simulink model "gm_DSBF"  (R2019b)
settings: Solver=FixedStepDiscrete  StartTime=0.0  StopTime=0.02  RelTol=1e-3
InitFcn:
  | sm_callback_init
StopFcn:
  | sm_callback_stop
undefined symbols (not defined in the file or in its folder): arraySize, arraySpacing, delayDataTypeFractionLength, delayDataTypeSign, delayDataTypeWordLength, mp, samplingRate, speedOfSound, upsampleFactor
libraries: hdlsllib x64, simulink x36, dspmlti4 x16, dsphdlfiltering x16
(part 2 of 5)

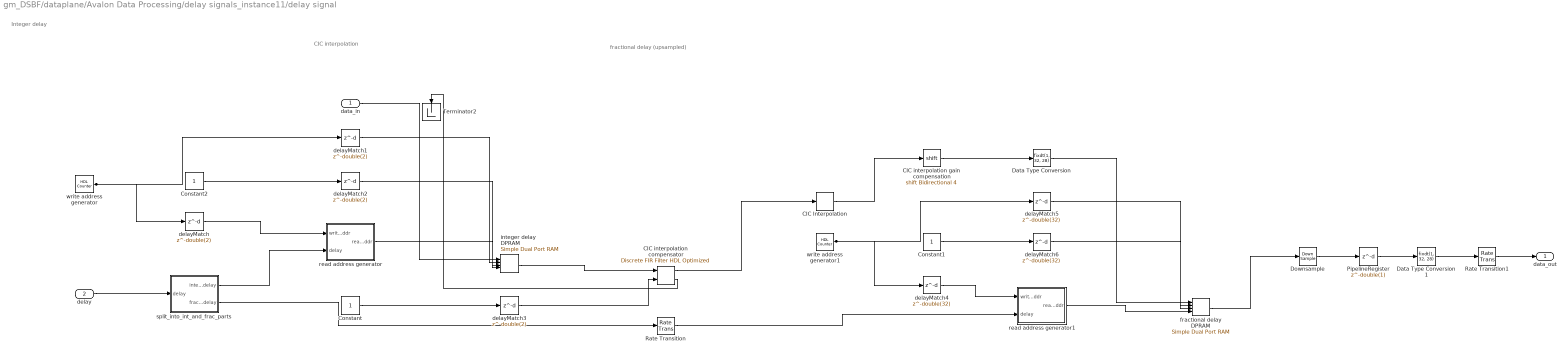
== system gm_DSBF/dataplane/Avalon Data Processing/delay signals_instance11/delay signal ==
  note: CIC interpolation
  note: Integer delay
  note: fractional delay (upsampled)
  data_in : Inport  OutDataTypeStr=fixdt(1, 32, 28)  PortDimensions=1  SampleTime=2.08333333333333e-05
  delay : Inport  Port=2  OutDataTypeStr=fixdt(1, 12, 6)  PortDimensions=1  SampleTime=2.08333333333333e-05
  CIC Interpolation : dspmlti4/CIC Interpolation  filtFrom=Filter object  filtobj=mp.cicInterpolator  ftype=Interpolator  R=mp.upsampleFactor  M=1  N=2  filterInternals=Full precision  BPS=[16 16 16 16]  FLPS=0  outputWordLength=32  outputFracLength=0  launchFVT=off  framing=Allow multirate processing  OutputFrames=off
      settings: SourceProductName=DSP System Toolbox  SourceProductBaseCode=DS
  CIC interpolation compensator : dsphdlfiltering/Discrete FIR Filter HDL Optimized  NumeratorSource=Property  Numerator=mp.cicInterpolatorCompensator.coeffs.Numerator  NumeratorPrototype=[]  FilterStructure=Direct form systolic  SerializationOption=Maximum number of multipliers  NumberOfCycles=2  NumberOfMultipliers=4  SimulateUsing=Code generation  roundingMode=Floor  overflowMode=off  CoefficientsDataTypeStr=fixdt(1,16)  CoefficientsMin=[]  CoefficientsMax=[]  OutputDataTypeStr=Inherit: Same word length as input  OutputMin=[]  OutputMax=[]  ResetInputPort=off  HDLGlobalReset=off
      settings: SourceProductName=DSP System Toolbox  SourceProductBaseCode=DS
  CIC interpolation gain compensation : ArithShift  BitShiftNumber=4  BinPtShiftNumber=double(0)
  Constant : Constant  OutDataTypeStr=boolean  SampleTime=-1
  Constant1 : Constant  OutDataTypeStr=boolean  SampleTime=-1
  Constant2 : Constant  OutDataTypeStr=boolean  SampleTime=-1
  Data Type Conversion : DataTypeConversion  OutDataTypeStr=fixdt(1, 32, 28)  SampleTime=1.30208333333333e-06
  Data Type Conversion1 : DataTypeConversion  OutDataTypeStr=fixdt(1, 32, 28)  SampleTime=2.08333333333333e-05
  Downsample : DownSample  N=double(16)  phase=double(0)  RateOptions=Allow multirate processing
  PipelineRegister : Delay  DelayLength=double(1)  InitialCondition=0  SampleTime=2.08333333333333e-05
  Rate Transition : RateTransition  InitialCondition=double(0)  OutPortSampleTimeOpt=Multiple of input port sample time  OutPortSampleTimeMultiple=1/16
  Rate Transition1 : RateTransition  InitialCondition=double(0)  OutPortSampleTimeOpt=Multiple of input port sample time  OutPortSampleTimeMultiple=1/2048
  Terminator2 : Terminator
  delayMatch{,1..3} (4 alike) : Delay  DelayLength=double(2)  InitialCondition=0  SampleTime=2.08333333333333e-05
  delayMatch4 : Delay  DelayLength=double(32)  InitialCondition=0  SampleTime=1.30208333333333e-06
  delayMatch5 : Delay  DelayLength=double(32)  InitialCondition=0  SampleTime=1.30208333333333e-06
  delayMatch6 : Delay  DelayLength=double(32)  InitialCondition=0  SampleTime=1.30208333333333e-06
  fractional delay DPRAM : hdlsllib/HDL RAMs/Simple Dual Port RAM  ram_size=mp.fractionalDelayAddrSize
      settings: SourceProductName=Simulink  SourceProductBaseCode=SL
  integer delay DPRAM : hdlsllib/HDL RAMs/Simple Dual Port RAM  ram_size=mp.integerDelayAddrSize
      settings: SourceProductName=Simulink  SourceProductBaseCode=SL
  read address generator : Subsystem
  read address generator1 : Subsystem
  split_into_int_and_frac_parts : Subsystem
  write address generator : hdlsllib/Sources/HDL Counter  CountType=Count limited  CountInit=double(0)  CountStep=double(1)  CountMax=double(63)  CountFromType=Initial value  CountFrom=double(0)  CountResetPort=off  CountLoadPort=off  CountEnbPort=off  CountDirPort=off  CountDataType=Unsigned  CountWordLen=6  CountFracLen=0  CountSampTime=2.08333333333333e-05
      settings: SourceProductName=Simulink
  write address generator1 : hdlsllib/Sources/HDL Counter  CountType=Count limited  CountInit=double(0)  CountStep=double(1)  CountMax=double(63)  CountFromType=Initial value  CountFrom=double(0)  CountResetPort=off  CountLoadPort=off  CountEnbPort=off  CountDirPort=off  CountDataType=Unsigned  CountWordLen=6  CountFracLen=0  CountSampTime=1.30208333333333e-06
      settings: SourceProductName=Simulink
  data_out : Outport  VectorParamsAs1DForOutWhenUnconnected=off
  wires:
  Downsample/1 -> PipelineRegister/1
  CIC interpolation gain compensation/1 -> Data Type Conversion/1
  split_into_int_and_frac_parts/1(integer_delay) -> read address generator/2(delay)
  Constant1/1 -> delayMatch6/1
  write address generator1/1 -> delayMatch4/1, delayMatch5/1
  delayMatch5/1 -> fractional delay DPRAM/2
  Constant/1 -> delayMatch3/1
  Constant2/1 -> delayMatch2/1
  write address generator/1 -> delayMatch/1, delayMatch1/1
  delayMatch1/1 -> integer delay DPRAM/2
  delay/1 -> split_into_int_and_frac_parts/1(delay)
  data_in/1 -> integer delay DPRAM/1
  delayMatch3/1 -> CIC interpolation compensator/2
  delayMatch6/1 -> fractional delay DPRAM/3
  delayMatch2/1 -> integer delay DPRAM/3
  Data Type Conversion/1 -> fractional delay DPRAM/1
  Data Type Conversion1/1 -> Rate Transition1/1
  split_into_int_and_frac_parts/2(fractional_delay) -> Rate Transition/1
  read address generator/1(read_addr) -> integer delay DPRAM/4
  read address generator1/1(read_addr) -> fractional delay DPRAM/4
  CIC Interpolation/1 -> CIC interpolation gain compensation/1
  CIC interpolation compensator/2 -> Terminator2/1
  CIC interpolation compensator/1 -> CIC Interpolation/1
  PipelineRegister/1 -> Data Type Conversion1/1
  Rate Transition/1 -> read address generator1/2(delay)
  Rate Transition1/1 -> data_out/1
  fractional delay DPRAM/1 -> Downsample/1
  integer delay DPRAM/1 -> CIC interpolation compensator/1
  delayMatch/1 -> read address generator/1(write_addr)
  delayMatch4/1 -> read address generator1/1(write_addr)

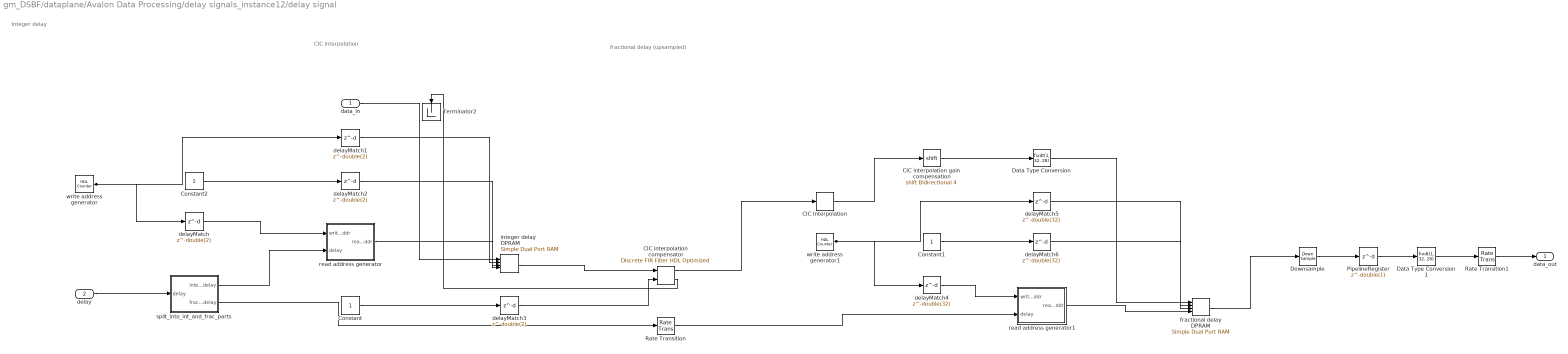
== system gm_DSBF/dataplane/Avalon Data Processing/delay signals_instance12/delay signal ==
  note: CIC interpolation
  note: Integer delay
  note: fractional delay (upsampled)
  data_in : Inport  OutDataTypeStr=fixdt(1, 32, 28)  PortDimensions=1  SampleTime=2.08333333333333e-05
  delay : Inport  Port=2  OutDataTypeStr=fixdt(1, 12, 6)  PortDimensions=1  SampleTime=2.08333333333333e-05
  CIC Interpolation : dspmlti4/CIC Interpolation  filtFrom=Filter object  filtobj=mp.cicInterpolator  ftype=Interpolator  R=mp.upsampleFactor  M=1  N=2  filterInternals=Full precision  BPS=[16 16 16 16]  FLPS=0  outputWordLength=32  outputFracLength=0  launchFVT=off  framing=Allow multirate processing  OutputFrames=off
      settings: SourceProductName=DSP System Toolbox  SourceProductBaseCode=DS
  CIC interpolation compensator : dsphdlfiltering/Discrete FIR Filter HDL Optimized  NumeratorSource=Property  Numerator=mp.cicInterpolatorCompensator.coeffs.Numerator  NumeratorPrototype=[]  FilterStructure=Direct form systolic  SerializationOption=Maximum number of multipliers  NumberOfCycles=2  NumberOfMultipliers=4  SimulateUsing=Code generation  roundingMode=Floor  overflowMode=off  CoefficientsDataTypeStr=fixdt(1,16)  CoefficientsMin=[]  CoefficientsMax=[]  OutputDataTypeStr=Inherit: Same word length as input  OutputMin=[]  OutputMax=[]  ResetInputPort=off  HDLGlobalReset=off
      settings: SourceProductName=DSP System Toolbox  SourceProductBaseCode=DS
  CIC interpolation gain compensation : ArithShift  BitShiftNumber=4  BinPtShiftNumber=double(0)
  Constant : Constant  OutDataTypeStr=boolean  SampleTime=-1
  Constant1 : Constant  OutDataTypeStr=boolean  SampleTime=-1
  Constant2 : Constant  OutDataTypeStr=boolean  SampleTime=-1
  Data Type Conversion : DataTypeConversion  OutDataTypeStr=fixdt(1, 32, 28)  SampleTime=1.30208333333333e-06
  Data Type Conversion1 : DataTypeConversion  OutDataTypeStr=fixdt(1, 32, 28)  SampleTime=2.08333333333333e-05
  Downsample : DownSample  N=double(16)  phase=double(0)  RateOptions=Allow multirate processing
  PipelineRegister : Delay  DelayLength=double(1)  InitialCondition=0  SampleTime=2.08333333333333e-05
  Rate Transition : RateTransition  InitialCondition=double(0)  OutPortSampleTimeOpt=Multiple of input port sample time  OutPortSampleTimeMultiple=1/16
  Rate Transition1 : RateTransition  InitialCondition=double(0)  OutPortSampleTimeOpt=Multiple of input port sample time  OutPortSampleTimeMultiple=1/2048
  Terminator2 : Terminator
  delayMatch{,1..3} (4 alike) : Delay  DelayLength=double(2)  InitialCondition=0  SampleTime=2.08333333333333e-05
  delayMatch4 : Delay  DelayLength=double(32)  InitialCondition=0  SampleTime=1.30208333333333e-06
  delayMatch5 : Delay  DelayLength=double(32)  InitialCondition=0  SampleTime=1.30208333333333e-06
  delayMatch6 : Delay  DelayLength=double(32)  InitialCondition=0  SampleTime=1.30208333333333e-06
  fractional delay DPRAM : hdlsllib/HDL RAMs/Simple Dual Port RAM  ram_size=mp.fractionalDelayAddrSize
      settings: SourceProductName=Simulink  SourceProductBaseCode=SL
  integer delay DPRAM : hdlsllib/HDL RAMs/Simple Dual Port RAM  ram_size=mp.integerDelayAddrSize
      settings: SourceProductName=Simulink  SourceProductBaseCode=SL
  read address generator : Subsystem
  read address generator1 : Subsystem
  split_into_int_and_frac_parts : Subsystem
  write address generator : hdlsllib/Sources/HDL Counter  CountType=Count limited  CountInit=double(0)  CountStep=double(1)  CountMax=double(63)  CountFromType=Initial value  CountFrom=double(0)  CountResetPort=off  CountLoadPort=off  CountEnbPort=off  CountDirPort=off  CountDataType=Unsigned  CountWordLen=6  CountFracLen=0  CountSampTime=2.08333333333333e-05
      settings: SourceProductName=Simulink
  write address generator1 : hdlsllib/Sources/HDL Counter  CountType=Count limited  CountInit=double(0)  CountStep=double(1)  CountMax=double(63)  CountFromType=Initial value  CountFrom=double(0)  CountResetPort=off  CountLoadPort=off  CountEnbPort=off  CountDirPort=off  CountDataType=Unsigned  CountWordLen=6  CountFracLen=0  CountSampTime=1.30208333333333e-06
      settings: SourceProductName=Simulink
  data_out : Outport  VectorParamsAs1DForOutWhenUnconnected=off
  wires:
  Downsample/1 -> PipelineRegister/1
  CIC interpolation gain compensation/1 -> Data Type Conversion/1
  split_into_int_and_frac_parts/1(integer_delay) -> read address generator/2(delay)
  Constant1/1 -> delayMatch6/1
  write address generator1/1 -> delayMatch4/1, delayMatch5/1
  delayMatch5/1 -> fractional delay DPRAM/2
  Constant/1 -> delayMatch3/1
  Constant2/1 -> delayMatch2/1
  write address generator/1 -> delayMatch/1, delayMatch1/1
  delayMatch1/1 -> integer delay DPRAM/2
  delay/1 -> split_into_int_and_frac_parts/1(delay)
  data_in/1 -> integer delay DPRAM/1
  delayMatch3/1 -> CIC interpolation compensator/2
  delayMatch6/1 -> fractional delay DPRAM/3
  delayMatch2/1 -> integer delay DPRAM/3
  Data Type Conversion/1 -> fractional delay DPRAM/1
  Data Type Conversion1/1 -> Rate Transition1/1
  split_into_int_and_frac_parts/2(fractional_delay) -> Rate Transition/1
  read address generator/1(read_addr) -> integer delay DPRAM/4
  read address generator1/1(read_addr) -> fractional delay DPRAM/4
  CIC Interpolation/1 -> CIC interpolation gain compensation/1
  CIC interpolation compensator/2 -> Terminator2/1
  CIC interpolation compensator/1 -> CIC Interpolation/1
  PipelineRegister/1 -> Data Type Conversion1/1
  Rate Transition/1 -> read address generator1/2(delay)
  Rate Transition1/1 -> data_out/1
  fractional delay DPRAM/1 -> Downsample/1
  integer delay DPRAM/1 -> CIC interpolation compensator/1
  delayMatch/1 -> read address generator/1(write_addr)
  delayMatch4/1 -> read address generator1/1(write_addr)

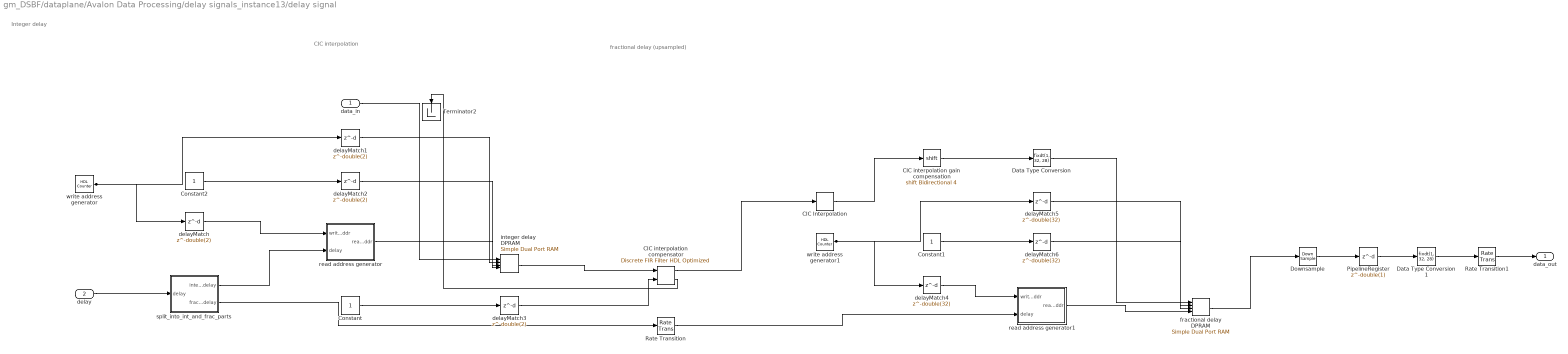
== system gm_DSBF/dataplane/Avalon Data Processing/delay signals_instance13/delay signal ==
  note: CIC interpolation
  note: Integer delay
  note: fractional delay (upsampled)
  data_in : Inport  OutDataTypeStr=fixdt(1, 32, 28)  PortDimensions=1  SampleTime=2.08333333333333e-05
  delay : Inport  Port=2  OutDataTypeStr=fixdt(1, 12, 6)  PortDimensions=1  SampleTime=2.08333333333333e-05
  CIC Interpolation : dspmlti4/CIC Interpolation  filtFrom=Filter object  filtobj=mp.cicInterpolator  ftype=Interpolator  R=mp.upsampleFactor  M=1  N=2  filterInternals=Full precision  BPS=[16 16 16 16]  FLPS=0  outputWordLength=32  outputFracLength=0  launchFVT=off  framing=Allow multirate processing  OutputFrames=off
      settings: SourceProductName=DSP System Toolbox  SourceProductBaseCode=DS
  CIC interpolation compensator : dsphdlfiltering/Discrete FIR Filter HDL Optimized  NumeratorSource=Property  Numerator=mp.cicInterpolatorCompensator.coeffs.Numerator  NumeratorPrototype=[]  FilterStructure=Direct form systolic  SerializationOption=Maximum number of multipliers  NumberOfCycles=2  NumberOfMultipliers=4  SimulateUsing=Code generation  roundingMode=Floor  overflowMode=off  CoefficientsDataTypeStr=fixdt(1,16)  CoefficientsMin=[]  CoefficientsMax=[]  OutputDataTypeStr=Inherit: Same word length as input  OutputMin=[]  OutputMax=[]  ResetInputPort=off  HDLGlobalReset=off
      settings: SourceProductName=DSP System Toolbox  SourceProductBaseCode=DS
  CIC interpolation gain compensation : ArithShift  BitShiftNumber=4  BinPtShiftNumber=double(0)
  Constant : Constant  OutDataTypeStr=boolean  SampleTime=-1
  Constant1 : Constant  OutDataTypeStr=boolean  SampleTime=-1
  Constant2 : Constant  OutDataTypeStr=boolean  SampleTime=-1
  Data Type Conversion : DataTypeConversion  OutDataTypeStr=fixdt(1, 32, 28)  SampleTime=1.30208333333333e-06
  Data Type Conversion1 : DataTypeConversion  OutDataTypeStr=fixdt(1, 32, 28)  SampleTime=2.08333333333333e-05
  Downsample : DownSample  N=double(16)  phase=double(0)  RateOptions=Allow multirate processing
  PipelineRegister : Delay  DelayLength=double(1)  InitialCondition=0  SampleTime=2.08333333333333e-05
  Rate Transition : RateTransition  InitialCondition=double(0)  OutPortSampleTimeOpt=Multiple of input port sample time  OutPortSampleTimeMultiple=1/16
  Rate Transition1 : RateTransition  InitialCondition=double(0)  OutPortSampleTimeOpt=Multiple of input port sample time  OutPortSampleTimeMultiple=1/2048
  Terminator2 : Terminator
  delayMatch{,1..3} (4 alike) : Delay  DelayLength=double(2)  InitialCondition=0  SampleTime=2.08333333333333e-05
  delayMatch4 : Delay  DelayLength=double(32)  InitialCondition=0  SampleTime=1.30208333333333e-06
  delayMatch5 : Delay  DelayLength=double(32)  InitialCondition=0  SampleTime=1.30208333333333e-06
  delayMatch6 : Delay  DelayLength=double(32)  InitialCondition=0  SampleTime=1.30208333333333e-06
  fractional delay DPRAM : hdlsllib/HDL RAMs/Simple Dual Port RAM  ram_size=mp.fractionalDelayAddrSize
      settings: SourceProductName=Simulink  SourceProductBaseCode=SL
  integer delay DPRAM : hdlsllib/HDL RAMs/Simple Dual Port RAM  ram_size=mp.integerDelayAddrSize
      settings: SourceProductName=Simulink  SourceProductBaseCode=SL
  read address generator : Subsystem
  read address generator1 : Subsystem
  split_into_int_and_frac_parts : Subsystem
  write address generator : hdlsllib/Sources/HDL Counter  CountType=Count limited  CountInit=double(0)  CountStep=double(1)  CountMax=double(63)  CountFromType=Initial value  CountFrom=double(0)  CountResetPort=off  CountLoadPort=off  CountEnbPort=off  CountDirPort=off  CountDataType=Unsigned  CountWordLen=6  CountFracLen=0  CountSampTime=2.08333333333333e-05
      settings: SourceProductName=Simulink
  write address generator1 : hdlsllib/Sources/HDL Counter  CountType=Count limited  CountInit=double(0)  CountStep=double(1)  CountMax=double(63)  CountFromType=Initial value  CountFrom=double(0)  CountResetPort=off  CountLoadPort=off  CountEnbPort=off  CountDirPort=off  CountDataType=Unsigned  CountWordLen=6  CountFracLen=0  CountSampTime=1.30208333333333e-06
      settings: SourceProductName=Simulink
  data_out : Outport  VectorParamsAs1DForOutWhenUnconnected=off
  wires:
  Downsample/1 -> PipelineRegister/1
  CIC interpolation gain compensation/1 -> Data Type Conversion/1
  split_into_int_and_frac_parts/1(integer_delay) -> read address generator/2(delay)
  Constant1/1 -> delayMatch6/1
  write address generator1/1 -> delayMatch4/1, delayMatch5/1
  delayMatch5/1 -> fractional delay DPRAM/2
  Constant/1 -> delayMatch3/1
  Constant2/1 -> delayMatch2/1
  write address generator/1 -> delayMatch/1, delayMatch1/1
  delayMatch1/1 -> integer delay DPRAM/2
  delay/1 -> split_into_int_and_frac_parts/1(delay)
  data_in/1 -> integer delay DPRAM/1
  delayMatch3/1 -> CIC interpolation compensator/2
  delayMatch6/1 -> fractional delay DPRAM/3
  delayMatch2/1 -> integer delay DPRAM/3
  Data Type Conversion/1 -> fractional delay DPRAM/1
  Data Type Conversion1/1 -> Rate Transition1/1
  split_into_int_and_frac_parts/2(fractional_delay) -> Rate Transition/1
  read address generator/1(read_addr) -> integer delay DPRAM/4
  read address generator1/1(read_addr) -> fractional delay DPRAM/4
  CIC Interpolation/1 -> CIC interpolation gain compensation/1
  CIC interpolation compensator/2 -> Terminator2/1
  CIC interpolation compensator/1 -> CIC Interpolation/1
  PipelineRegister/1 -> Data Type Conversion1/1
  Rate Transition/1 -> read address generator1/2(delay)
  Rate Transition1/1 -> data_out/1
  fractional delay DPRAM/1 -> Downsample/1
  integer delay DPRAM/1 -> CIC interpolation compensator/1
  delayMatch/1 -> read address generator/1(write_addr)
  delayMatch4/1 -> read address generator1/1(write_addr)

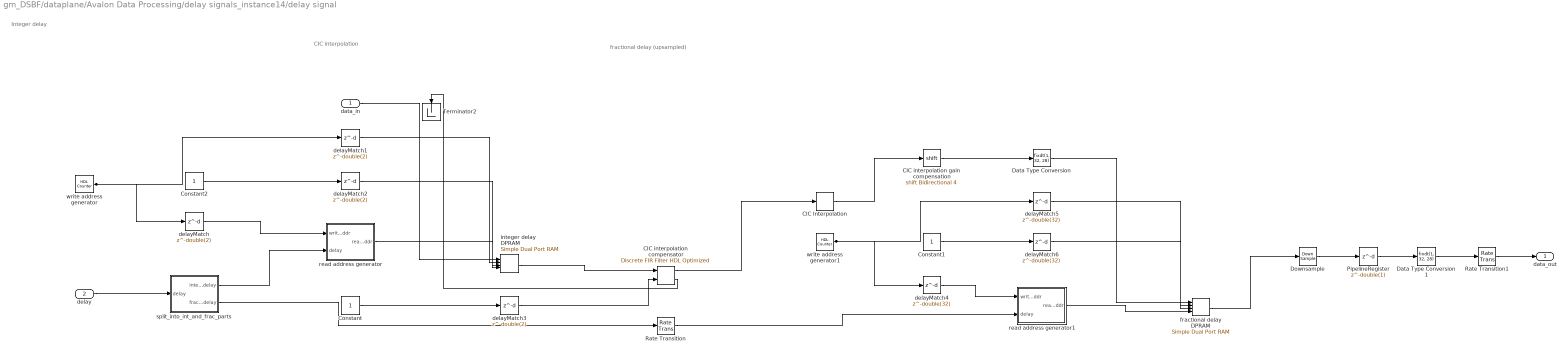
== system gm_DSBF/dataplane/Avalon Data Processing/delay signals_instance14/delay signal ==
  note: CIC interpolation
  note: Integer delay
  note: fractional delay (upsampled)
  data_in : Inport  OutDataTypeStr=fixdt(1, 32, 28)  PortDimensions=1  SampleTime=2.08333333333333e-05
  delay : Inport  Port=2  OutDataTypeStr=fixdt(1, 12, 6)  PortDimensions=1  SampleTime=2.08333333333333e-05
  CIC Interpolation : dspmlti4/CIC Interpolation  filtFrom=Filter object  filtobj=mp.cicInterpolator  ftype=Interpolator  R=mp.upsampleFactor  M=1  N=2  filterInternals=Full precision  BPS=[16 16 16 16]  FLPS=0  outputWordLength=32  outputFracLength=0  launchFVT=off  framing=Allow multirate processing  OutputFrames=off
      settings: SourceProductName=DSP System Toolbox  SourceProductBaseCode=DS
  CIC interpolation compensator : dsphdlfiltering/Discrete FIR Filter HDL Optimized  NumeratorSource=Property  Numerator=mp.cicInterpolatorCompensator.coeffs.Numerator  NumeratorPrototype=[]  FilterStructure=Direct form systolic  SerializationOption=Maximum number of multipliers  NumberOfCycles=2  NumberOfMultipliers=4  SimulateUsing=Code generation  roundingMode=Floor  overflowMode=off  CoefficientsDataTypeStr=fixdt(1,16)  CoefficientsMin=[]  CoefficientsMax=[]  OutputDataTypeStr=Inherit: Same word length as input  OutputMin=[]  OutputMax=[]  ResetInputPort=off  HDLGlobalReset=off
      settings: SourceProductName=DSP System Toolbox  SourceProductBaseCode=DS
  CIC interpolation gain compensation : ArithShift  BitShiftNumber=4  BinPtShiftNumber=double(0)
  Constant : Constant  OutDataTypeStr=boolean  SampleTime=-1
  Constant1 : Constant  OutDataTypeStr=boolean  SampleTime=-1
  Constant2 : Constant  OutDataTypeStr=boolean  SampleTime=-1
  Data Type Conversion : DataTypeConversion  OutDataTypeStr=fixdt(1, 32, 28)  SampleTime=1.30208333333333e-06
  Data Type Conversion1 : DataTypeConversion  OutDataTypeStr=fixdt(1, 32, 28)  SampleTime=2.08333333333333e-05
  Downsample : DownSample  N=double(16)  phase=double(0)  RateOptions=Allow multirate processing
  PipelineRegister : Delay  DelayLength=double(1)  InitialCondition=0  SampleTime=2.08333333333333e-05
  Rate Transition : RateTransition  InitialCondition=double(0)  OutPortSampleTimeOpt=Multiple of input port sample time  OutPortSampleTimeMultiple=1/16
  Rate Transition1 : RateTransition  InitialCondition=double(0)  OutPortSampleTimeOpt=Multiple of input port sample time  OutPortSampleTimeMultiple=1/2048
  Terminator2 : Terminator
  delayMatch{,1..3} (4 alike) : Delay  DelayLength=double(2)  InitialCondition=0  SampleTime=2.08333333333333e-05
  delayMatch4 : Delay  DelayLength=double(32)  InitialCondition=0  SampleTime=1.30208333333333e-06
  delayMatch5 : Delay  DelayLength=double(32)  InitialCondition=0  SampleTime=1.30208333333333e-06
  delayMatch6 : Delay  DelayLength=double(32)  InitialCondition=0  SampleTime=1.30208333333333e-06
  fractional delay DPRAM : hdlsllib/HDL RAMs/Simple Dual Port RAM  ram_size=mp.fractionalDelayAddrSize
      settings: SourceProductName=Simulink  SourceProductBaseCode=SL
  integer delay DPRAM : hdlsllib/HDL RAMs/Simple Dual Port RAM  ram_size=mp.integerDelayAddrSize
      settings: SourceProductName=Simulink  SourceProductBaseCode=SL
  read address generator : Subsystem
  read address generator1 : Subsystem
  split_into_int_and_frac_parts : Subsystem
  write address generator : hdlsllib/Sources/HDL Counter  CountType=Count limited  CountInit=double(0)  CountStep=double(1)  CountMax=double(63)  CountFromType=Initial value  CountFrom=double(0)  CountResetPort=off  CountLoadPort=off  CountEnbPort=off  CountDirPort=off  CountDataType=Unsigned  CountWordLen=6  CountFracLen=0  CountSampTime=2.08333333333333e-05
      settings: SourceProductName=Simulink
  write address generator1 : hdlsllib/Sources/HDL Counter  CountType=Count limited  CountInit=double(0)  CountStep=double(1)  CountMax=double(63)  CountFromType=Initial value  CountFrom=double(0)  CountResetPort=off  CountLoadPort=off  CountEnbPort=off  CountDirPort=off  CountDataType=Unsigned  CountWordLen=6  CountFracLen=0  CountSampTime=1.30208333333333e-06
      settings: SourceProductName=Simulink
  data_out : Outport  VectorParamsAs1DForOutWhenUnconnected=off
  wires:
  Downsample/1 -> PipelineRegister/1
  CIC interpolation gain compensation/1 -> Data Type Conversion/1
  split_into_int_and_frac_parts/1(integer_delay) -> read address generator/2(delay)
  Constant1/1 -> delayMatch6/1
  write address generator1/1 -> delayMatch4/1, delayMatch5/1
  delayMatch5/1 -> fractional delay DPRAM/2
  Constant/1 -> delayMatch3/1
  Constant2/1 -> delayMatch2/1
  write address generator/1 -> delayMatch/1, delayMatch1/1
  delayMatch1/1 -> integer delay DPRAM/2
  delay/1 -> split_into_int_and_frac_parts/1(delay)
  data_in/1 -> integer delay DPRAM/1
  delayMatch3/1 -> CIC interpolation compensator/2
  delayMatch6/1 -> fractional delay DPRAM/3
  delayMatch2/1 -> integer delay DPRAM/3
  Data Type Conversion/1 -> fractional delay DPRAM/1
  Data Type Conversion1/1 -> Rate Transition1/1
  split_into_int_and_frac_parts/2(fractional_delay) -> Rate Transition/1
  read address generator/1(read_addr) -> integer delay DPRAM/4
  read address generator1/1(read_addr) -> fractional delay DPRAM/4
  CIC Interpolation/1 -> CIC interpolation gain compensation/1
  CIC interpolation compensator/2 -> Terminator2/1
  CIC interpolation compensator/1 -> CIC Interpolation/1
  PipelineRegister/1 -> Data Type Conversion1/1
  Rate Transition/1 -> read address generator1/2(delay)
  Rate Transition1/1 -> data_out/1
  fractional delay DPRAM/1 -> Downsample/1
  integer delay DPRAM/1 -> CIC interpolation compensator/1
  delayMatch/1 -> read address generator/1(write_addr)
  delayMatch4/1 -> read address generator1/1(write_addr)

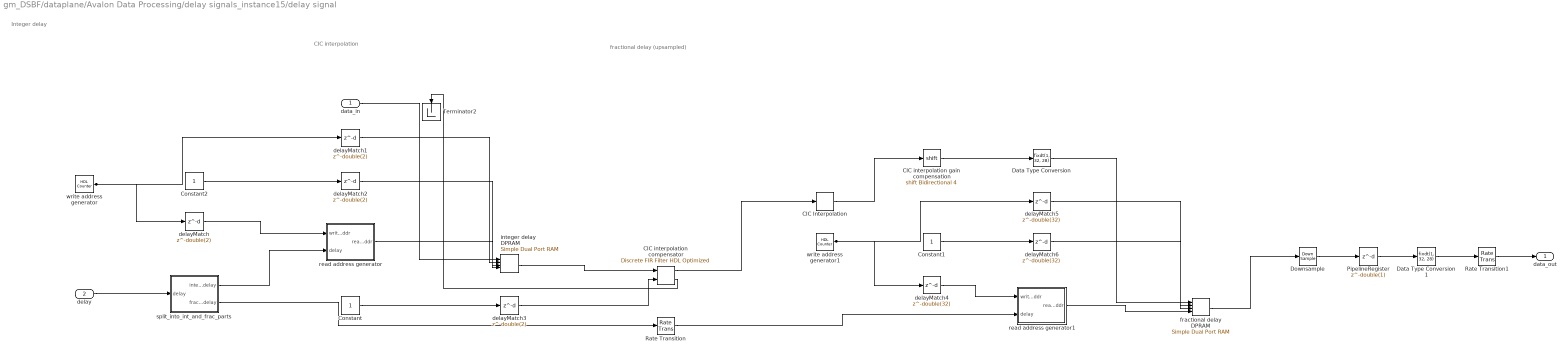
== system gm_DSBF/dataplane/Avalon Data Processing/delay signals_instance15/delay signal ==
  note: CIC interpolation
  note: Integer delay
  note: fractional delay (upsampled)
  data_in : Inport  OutDataTypeStr=fixdt(1, 32, 28)  PortDimensions=1  SampleTime=2.08333333333333e-05
  delay : Inport  Port=2  OutDataTypeStr=fixdt(1, 12, 6)  PortDimensions=1  SampleTime=2.08333333333333e-05
  CIC Interpolation : dspmlti4/CIC Interpolation  filtFrom=Filter object  filtobj=mp.cicInterpolator  ftype=Interpolator  R=mp.upsampleFactor  M=1  N=2  filterInternals=Full precision  BPS=[16 16 16 16]  FLPS=0  outputWordLength=32  outputFracLength=0  launchFVT=off  framing=Allow multirate processing  OutputFrames=off
      settings: SourceProductName=DSP System Toolbox  SourceProductBaseCode=DS
  CIC interpolation compensator : dsphdlfiltering/Discrete FIR Filter HDL Optimized  NumeratorSource=Property  Numerator=mp.cicInterpolatorCompensator.coeffs.Numerator  NumeratorPrototype=[]  FilterStructure=Direct form systolic  SerializationOption=Maximum number of multipliers  NumberOfCycles=2  NumberOfMultipliers=4  SimulateUsing=Code generation  roundingMode=Floor  overflowMode=off  CoefficientsDataTypeStr=fixdt(1,16)  CoefficientsMin=[]  CoefficientsMax=[]  OutputDataTypeStr=Inherit: Same word length as input  OutputMin=[]  OutputMax=[]  ResetInputPort=off  HDLGlobalReset=off
      settings: SourceProductName=DSP System Toolbox  SourceProductBaseCode=DS
  CIC interpolation gain compensation : ArithShift  BitShiftNumber=4  BinPtShiftNumber=double(0)
  Constant : Constant  OutDataTypeStr=boolean  SampleTime=-1
  Constant1 : Constant  OutDataTypeStr=boolean  SampleTime=-1
  Constant2 : Constant  OutDataTypeStr=boolean  SampleTime=-1
  Data Type Conversion : DataTypeConversion  OutDataTypeStr=fixdt(1, 32, 28)  SampleTime=1.30208333333333e-06
  Data Type Conversion1 : DataTypeConversion  OutDataTypeStr=fixdt(1, 32, 28)  SampleTime=2.08333333333333e-05
  Downsample : DownSample  N=double(16)  phase=double(0)  RateOptions=Allow multirate processing
  PipelineRegister : Delay  DelayLength=double(1)  InitialCondition=0  SampleTime=2.08333333333333e-05
  Rate Transition : RateTransition  InitialCondition=double(0)  OutPortSampleTimeOpt=Multiple of input port sample time  OutPortSampleTimeMultiple=1/16
  Rate Transition1 : RateTransition  InitialCondition=double(0)  OutPortSampleTimeOpt=Multiple of input port sample time  OutPortSampleTimeMultiple=1/2048
  Terminator2 : Terminator
  delayMatch{,1..3} (4 alike) : Delay  DelayLength=double(2)  InitialCondition=0  SampleTime=2.08333333333333e-05
  delayMatch4 : Delay  DelayLength=double(32)  InitialCondition=0  SampleTime=1.30208333333333e-06
  delayMatch5 : Delay  DelayLength=double(32)  InitialCondition=0  SampleTime=1.30208333333333e-06
  delayMatch6 : Delay  DelayLength=double(32)  InitialCondition=0  SampleTime=1.30208333333333e-06
  fractional delay DPRAM : hdlsllib/HDL RAMs/Simple Dual Port RAM  ram_size=mp.fractionalDelayAddrSize
      settings: SourceProductName=Simulink  SourceProductBaseCode=SL
  integer delay DPRAM : hdlsllib/HDL RAMs/Simple Dual Port RAM  ram_size=mp.integerDelayAddrSize
      settings: SourceProductName=Simulink  SourceProductBaseCode=SL
  read address generator : Subsystem
  read address generator1 : Subsystem
  split_into_int_and_frac_parts : Subsystem
  write address generator : hdlsllib/Sources/HDL Counter  CountType=Count limited  CountInit=double(0)  CountStep=double(1)  CountMax=double(63)  CountFromType=Initial value  CountFrom=double(0)  CountResetPort=off  CountLoadPort=off  CountEnbPort=off  CountDirPort=off  CountDataType=Unsigned  CountWordLen=6  CountFracLen=0  CountSampTime=2.08333333333333e-05
      settings: SourceProductName=Simulink
  write address generator1 : hdlsllib/Sources/HDL Counter  CountType=Count limited  CountInit=double(0)  CountStep=double(1)  CountMax=double(63)  CountFromType=Initial value  CountFrom=double(0)  CountResetPort=off  CountLoadPort=off  CountEnbPort=off  CountDirPort=off  CountDataType=Unsigned  CountWordLen=6  CountFracLen=0  CountSampTime=1.30208333333333e-06
      settings: SourceProductName=Simulink
  data_out : Outport  VectorParamsAs1DForOutWhenUnconnected=off
  wires:
  Downsample/1 -> PipelineRegister/1
  CIC interpolation gain compensation/1 -> Data Type Conversion/1
  split_into_int_and_frac_parts/1(integer_delay) -> read address generator/2(delay)
  Constant1/1 -> delayMatch6/1
  write address generator1/1 -> delayMatch4/1, delayMatch5/1
  delayMatch5/1 -> fractional delay DPRAM/2
  Constant/1 -> delayMatch3/1
  Constant2/1 -> delayMatch2/1
  write address generator/1 -> delayMatch/1, delayMatch1/1
  delayMatch1/1 -> integer delay DPRAM/2
  delay/1 -> split_into_int_and_frac_parts/1(delay)
  data_in/1 -> integer delay DPRAM/1
  delayMatch3/1 -> CIC interpolation compensator/2
  delayMatch6/1 -> fractional delay DPRAM/3
  delayMatch2/1 -> integer delay DPRAM/3
  Data Type Conversion/1 -> fractional delay DPRAM/1
  Data Type Conversion1/1 -> Rate Transition1/1
  split_into_int_and_frac_parts/2(fractional_delay) -> Rate Transition/1
  read address generator/1(read_addr) -> integer delay DPRAM/4
  read address generator1/1(read_addr) -> fractional delay DPRAM/4
  CIC Interpolation/1 -> CIC interpolation gain compensation/1
  CIC interpolation compensator/2 -> Terminator2/1
  CIC interpolation compensator/1 -> CIC Interpolation/1
  PipelineRegister/1 -> Data Type Conversion1/1
  Rate Transition/1 -> read address generator1/2(delay)
  Rate Transition1/1 -> data_out/1
  fractional delay DPRAM/1 -> Downsample/1
  integer delay DPRAM/1 -> CIC interpolation compensator/1
  delayMatch/1 -> read address generator/1(write_addr)
  delayMatch4/1 -> read address generator1/1(write_addr)

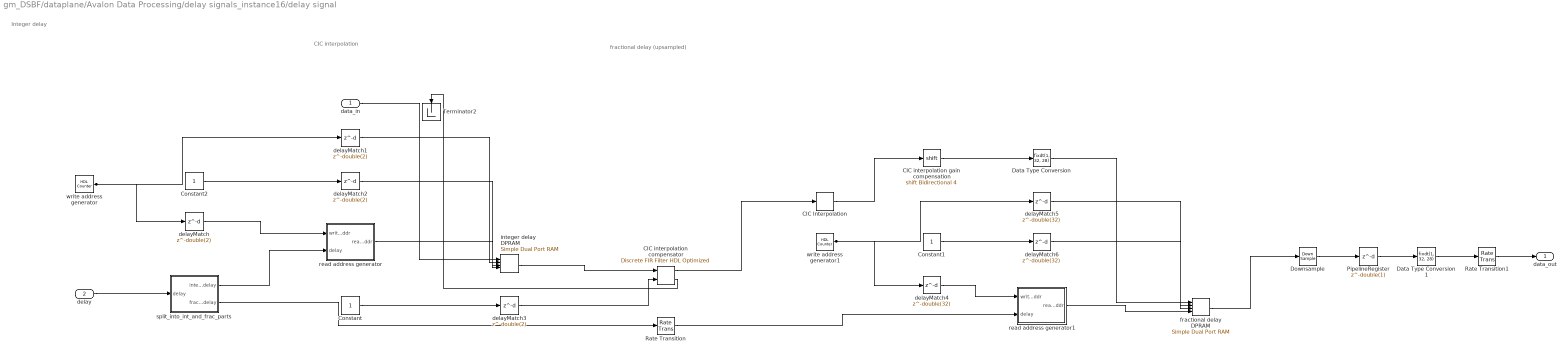
== system gm_DSBF/dataplane/Avalon Data Processing/delay signals_instance16/delay signal ==
  note: CIC interpolation
  note: Integer delay
  note: fractional delay (upsampled)
  data_in : Inport  OutDataTypeStr=fixdt(1, 32, 28)  PortDimensions=1  SampleTime=2.08333333333333e-05
  delay : Inport  Port=2  OutDataTypeStr=fixdt(1, 12, 6)  PortDimensions=1  SampleTime=2.08333333333333e-05
  CIC Interpolation : dspmlti4/CIC Interpolation  filtFrom=Filter object  filtobj=mp.cicInterpolator  ftype=Interpolator  R=mp.upsampleFactor  M=1  N=2  filterInternals=Full precision  BPS=[16 16 16 16]  FLPS=0  outputWordLength=32  outputFracLength=0  launchFVT=off  framing=Allow multirate processing  OutputFrames=off
      settings: SourceProductName=DSP System Toolbox  SourceProductBaseCode=DS
  CIC interpolation compensator : dsphdlfiltering/Discrete FIR Filter HDL Optimized  NumeratorSource=Property  Numerator=mp.cicInterpolatorCompensator.coeffs.Numerator  NumeratorPrototype=[]  FilterStructure=Direct form systolic  SerializationOption=Maximum number of multipliers  NumberOfCycles=2  NumberOfMultipliers=4  SimulateUsing=Code generation  roundingMode=Floor  overflowMode=off  CoefficientsDataTypeStr=fixdt(1,16)  CoefficientsMin=[]  CoefficientsMax=[]  OutputDataTypeStr=Inherit: Same word length as input  OutputMin=[]  OutputMax=[]  ResetInputPort=off  HDLGlobalReset=off
      settings: SourceProductName=DSP System Toolbox  SourceProductBaseCode=DS
  CIC interpolation gain compensation : ArithShift  BitShiftNumber=4  BinPtShiftNumber=double(0)
  Constant : Constant  OutDataTypeStr=boolean  SampleTime=-1
  Constant1 : Constant  OutDataTypeStr=boolean  SampleTime=-1
  Constant2 : Constant  OutDataTypeStr=boolean  SampleTime=-1
  Data Type Conversion : DataTypeConversion  OutDataTypeStr=fixdt(1, 32, 28)  SampleTime=1.30208333333333e-06
  Data Type Conversion1 : DataTypeConversion  OutDataTypeStr=fixdt(1, 32, 28)  SampleTime=2.08333333333333e-05
  Downsample : DownSample  N=double(16)  phase=double(0)  RateOptions=Allow multirate processing
  PipelineRegister : Delay  DelayLength=double(1)  InitialCondition=0  SampleTime=2.08333333333333e-05
  Rate Transition : RateTransition  InitialCondition=double(0)  OutPortSampleTimeOpt=Multiple of input port sample time  OutPortSampleTimeMultiple=1/16
  Rate Transition1 : RateTransition  InitialCondition=double(0)  OutPortSampleTimeOpt=Multiple of input port sample time  OutPortSampleTimeMultiple=1/2048
  Terminator2 : Terminator
  delayMatch{,1..3} (4 alike) : Delay  DelayLength=double(2)  InitialCondition=0  SampleTime=2.08333333333333e-05
  delayMatch4 : Delay  DelayLength=double(32)  InitialCondition=0  SampleTime=1.30208333333333e-06
  delayMatch5 : Delay  DelayLength=double(32)  InitialCondition=0  SampleTime=1.30208333333333e-06
  delayMatch6 : Delay  DelayLength=double(32)  InitialCondition=0  SampleTime=1.30208333333333e-06
  fractional delay DPRAM : hdlsllib/HDL RAMs/Simple Dual Port RAM  ram_size=mp.fractionalDelayAddrSize
      settings: SourceProductName=Simulink  SourceProductBaseCode=SL
  integer delay DPRAM : hdlsllib/HDL RAMs/Simple Dual Port RAM  ram_size=mp.integerDelayAddrSize
      settings: SourceProductName=Simulink  SourceProductBaseCode=SL
  read address generator : Subsystem
  read address generator1 : Subsystem
  split_into_int_and_frac_parts : Subsystem
  write address generator : hdlsllib/Sources/HDL Counter  CountType=Count limited  CountInit=double(0)  CountStep=double(1)  CountMax=double(63)  CountFromType=Initial value  CountFrom=double(0)  CountResetPort=off  CountLoadPort=off  CountEnbPort=off  CountDirPort=off  CountDataType=Unsigned  CountWordLen=6  CountFracLen=0  CountSampTime=2.08333333333333e-05
      settings: SourceProductName=Simulink
  write address generator1 : hdlsllib/Sources/HDL Counter  CountType=Count limited  CountInit=double(0)  CountStep=double(1)  CountMax=double(63)  CountFromType=Initial value  CountFrom=double(0)  CountResetPort=off  CountLoadPort=off  CountEnbPort=off  CountDirPort=off  CountDataType=Unsigned  CountWordLen=6  CountFracLen=0  CountSampTime=1.30208333333333e-06
      settings: SourceProductName=Simulink
  data_out : Outport  VectorParamsAs1DForOutWhenUnconnected=off
  wires:
  Downsample/1 -> PipelineRegister/1
  CIC interpolation gain compensation/1 -> Data Type Conversion/1
  split_into_int_and_frac_parts/1(integer_delay) -> read address generator/2(delay)
  Constant1/1 -> delayMatch6/1
  write address generator1/1 -> delayMatch4/1, delayMatch5/1
  delayMatch5/1 -> fractional delay DPRAM/2
  Constant/1 -> delayMatch3/1
  Constant2/1 -> delayMatch2/1
  write address generator/1 -> delayMatch/1, delayMatch1/1
  delayMatch1/1 -> integer delay DPRAM/2
  delay/1 -> split_into_int_and_frac_parts/1(delay)
  data_in/1 -> integer delay DPRAM/1
  delayMatch3/1 -> CIC interpolation compensator/2
  delayMatch6/1 -> fractional delay DPRAM/3
  delayMatch2/1 -> integer delay DPRAM/3
  Data Type Conversion/1 -> fractional delay DPRAM/1
  Data Type Conversion1/1 -> Rate Transition1/1
  split_into_int_and_frac_parts/2(fractional_delay) -> Rate Transition/1
  read address generator/1(read_addr) -> integer delay DPRAM/4
  read address generator1/1(read_addr) -> fractional delay DPRAM/4
  CIC Interpolation/1 -> CIC interpolation gain compensation/1
  CIC interpolation compensator/2 -> Terminator2/1
  CIC interpolation compensator/1 -> CIC Interpolation/1
  PipelineRegister/1 -> Data Type Conversion1/1
  Rate Transition/1 -> read address generator1/2(delay)
  Rate Transition1/1 -> data_out/1
  fractional delay DPRAM/1 -> Downsample/1
  integer delay DPRAM/1 -> CIC interpolation compensator/1
  delayMatch/1 -> read address generator/1(write_addr)
  delayMatch4/1 -> read address generator1/1(write_addr)

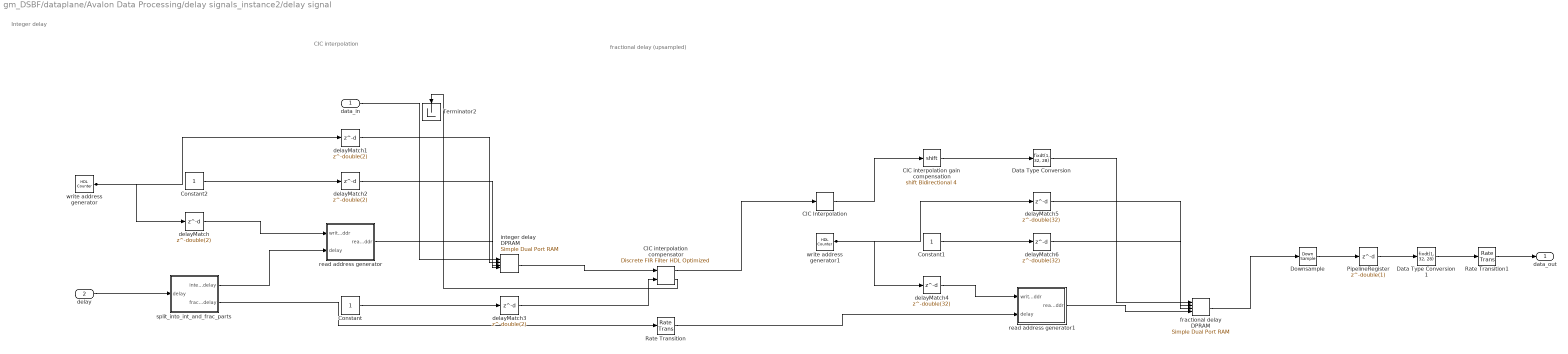
== system gm_DSBF/dataplane/Avalon Data Processing/delay signals_instance2/delay signal ==
  note: CIC interpolation
  note: Integer delay
  note: fractional delay (upsampled)
  data_in : Inport  OutDataTypeStr=fixdt(1, 32, 28)  PortDimensions=1  SampleTime=2.08333333333333e-05
  delay : Inport  Port=2  OutDataTypeStr=fixdt(1, 12, 6)  PortDimensions=1  SampleTime=2.08333333333333e-05
  CIC Interpolation : dspmlti4/CIC Interpolation  filtFrom=Filter object  filtobj=mp.cicInterpolator  ftype=Interpolator  R=mp.upsampleFactor  M=1  N=2  filterInternals=Full precision  BPS=[16 16 16 16]  FLPS=0  outputWordLength=32  outputFracLength=0  launchFVT=off  framing=Allow multirate processing  OutputFrames=off
      settings: SourceProductName=DSP System Toolbox  SourceProductBaseCode=DS
  CIC interpolation compensator : dsphdlfiltering/Discrete FIR Filter HDL Optimized  NumeratorSource=Property  Numerator=mp.cicInterpolatorCompensator.coeffs.Numerator  NumeratorPrototype=[]  FilterStructure=Direct form systolic  SerializationOption=Maximum number of multipliers  NumberOfCycles=2  NumberOfMultipliers=4  SimulateUsing=Code generation  roundingMode=Floor  overflowMode=off  CoefficientsDataTypeStr=fixdt(1,16)  CoefficientsMin=[]  CoefficientsMax=[]  OutputDataTypeStr=Inherit: Same word length as input  OutputMin=[]  OutputMax=[]  ResetInputPort=off  HDLGlobalReset=off
      settings: SourceProductName=DSP System Toolbox  SourceProductBaseCode=DS
  CIC interpolation gain compensation : ArithShift  BitShiftNumber=4  BinPtShiftNumber=double(0)
  Constant : Constant  OutDataTypeStr=boolean  SampleTime=-1
  Constant1 : Constant  OutDataTypeStr=boolean  SampleTime=-1
  Constant2 : Constant  OutDataTypeStr=boolean  SampleTime=-1
  Data Type Conversion : DataTypeConversion  OutDataTypeStr=fixdt(1, 32, 28)  SampleTime=1.30208333333333e-06
  Data Type Conversion1 : DataTypeConversion  OutDataTypeStr=fixdt(1, 32, 28)  SampleTime=2.08333333333333e-05
  Downsample : DownSample  N=double(16)  phase=double(0)  RateOptions=Allow multirate processing
  PipelineRegister : Delay  DelayLength=double(1)  InitialCondition=0  SampleTime=2.08333333333333e-05
  Rate Transition : RateTransition  InitialCondition=double(0)  OutPortSampleTimeOpt=Multiple of input port sample time  OutPortSampleTimeMultiple=1/16
  Rate Transition1 : RateTransition  InitialCondition=double(0)  OutPortSampleTimeOpt=Multiple of input port sample time  OutPortSampleTimeMultiple=1/2048
  Terminator2 : Terminator
  delayMatch{,1..3} (4 alike) : Delay  DelayLength=double(2)  InitialCondition=0  SampleTime=2.08333333333333e-05
  delayMatch4 : Delay  DelayLength=double(32)  InitialCondition=0  SampleTime=1.30208333333333e-06
  delayMatch5 : Delay  DelayLength=double(32)  InitialCondition=0  SampleTime=1.30208333333333e-06
  delayMatch6 : Delay  DelayLength=double(32)  InitialCondition=0  SampleTime=1.30208333333333e-06
  fractional delay DPRAM : hdlsllib/HDL RAMs/Simple Dual Port RAM  ram_size=mp.fractionalDelayAddrSize
      settings: SourceProductName=Simulink  SourceProductBaseCode=SL
  integer delay DPRAM : hdlsllib/HDL RAMs/Simple Dual Port RAM  ram_size=mp.integerDelayAddrSize
      settings: SourceProductName=Simulink  SourceProductBaseCode=SL
  read address generator : Subsystem
  read address generator1 : Subsystem
  split_into_int_and_frac_parts : Subsystem
  write address generator : hdlsllib/Sources/HDL Counter  CountType=Count limited  CountInit=double(0)  CountStep=double(1)  CountMax=double(63)  CountFromType=Initial value  CountFrom=double(0)  CountResetPort=off  CountLoadPort=off  CountEnbPort=off  CountDirPort=off  CountDataType=Unsigned  CountWordLen=6  CountFracLen=0  CountSampTime=2.08333333333333e-05
      settings: SourceProductName=Simulink
  write address generator1 : hdlsllib/Sources/HDL Counter  CountType=Count limited  CountInit=double(0)  CountStep=double(1)  CountMax=double(63)  CountFromType=Initial value  CountFrom=double(0)  CountResetPort=off  CountLoadPort=off  CountEnbPort=off  CountDirPort=off  CountDataType=Unsigned  CountWordLen=6  CountFracLen=0  CountSampTime=1.30208333333333e-06
      settings: SourceProductName=Simulink
  data_out : Outport  VectorParamsAs1DForOutWhenUnconnected=off
  wires:
  Downsample/1 -> PipelineRegister/1
  CIC interpolation gain compensation/1 -> Data Type Conversion/1
  split_into_int_and_frac_parts/1(integer_delay) -> read address generator/2(delay)
  Constant1/1 -> delayMatch6/1
  write address generator1/1 -> delayMatch4/1, delayMatch5/1
  delayMatch5/1 -> fractional delay DPRAM/2
  Constant/1 -> delayMatch3/1
  Constant2/1 -> delayMatch2/1
  write address generator/1 -> delayMatch/1, delayMatch1/1
  delayMatch1/1 -> integer delay DPRAM/2
  delay/1 -> split_into_int_and_frac_parts/1(delay)
  data_in/1 -> integer delay DPRAM/1
  delayMatch3/1 -> CIC interpolation compensator/2
  delayMatch6/1 -> fractional delay DPRAM/3
  delayMatch2/1 -> integer delay DPRAM/3
  Data Type Conversion/1 -> fractional delay DPRAM/1
  Data Type Conversion1/1 -> Rate Transition1/1
  split_into_int_and_frac_parts/2(fractional_delay) -> Rate Transition/1
  read address generator/1(read_addr) -> integer delay DPRAM/4
  read address generator1/1(read_addr) -> fractional delay DPRAM/4
  CIC Interpolation/1 -> CIC interpolation gain compensation/1
  CIC interpolation compensator/2 -> Terminator2/1
  CIC interpolation compensator/1 -> CIC Interpolation/1
  PipelineRegister/1 -> Data Type Conversion1/1
  Rate Transition/1 -> read address generator1/2(delay)
  Rate Transition1/1 -> data_out/1
  fractional delay DPRAM/1 -> Downsample/1
  integer delay DPRAM/1 -> CIC interpolation compensator/1
  delayMatch/1 -> read address generator/1(write_addr)
  delayMatch4/1 -> read address generator1/1(write_addr)

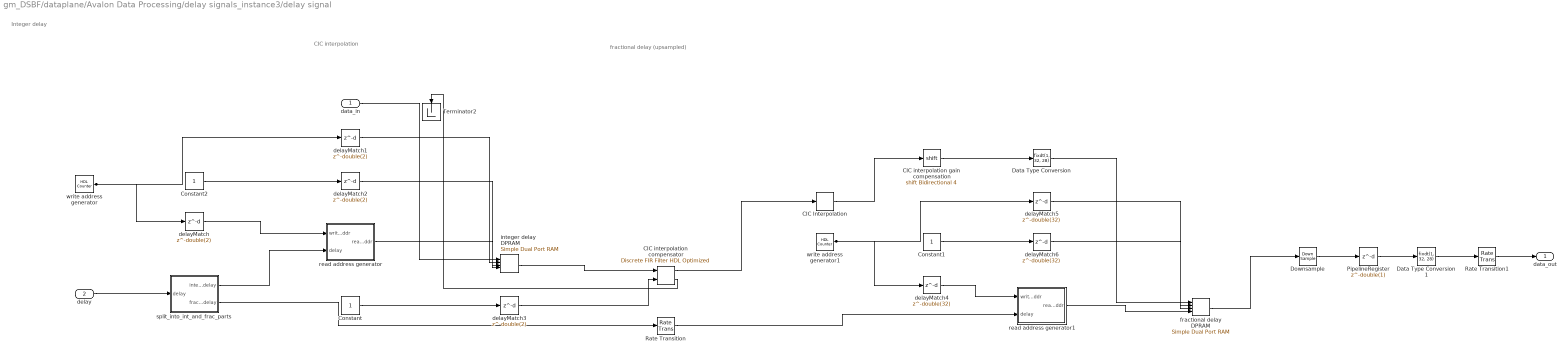
== system gm_DSBF/dataplane/Avalon Data Processing/delay signals_instance3/delay signal ==
  note: CIC interpolation
  note: Integer delay
  note: fractional delay (upsampled)
  data_in : Inport  OutDataTypeStr=fixdt(1, 32, 28)  PortDimensions=1  SampleTime=2.08333333333333e-05
  delay : Inport  Port=2  OutDataTypeStr=fixdt(1, 12, 6)  PortDimensions=1  SampleTime=2.08333333333333e-05
  CIC Interpolation : dspmlti4/CIC Interpolation  filtFrom=Filter object  filtobj=mp.cicInterpolator  ftype=Interpolator  R=mp.upsampleFactor  M=1  N=2  filterInternals=Full precision  BPS=[16 16 16 16]  FLPS=0  outputWordLength=32  outputFracLength=0  launchFVT=off  framing=Allow multirate processing  OutputFrames=off
      settings: SourceProductName=DSP System Toolbox  SourceProductBaseCode=DS
  CIC interpolation compensator : dsphdlfiltering/Discrete FIR Filter HDL Optimized  NumeratorSource=Property  Numerator=mp.cicInterpolatorCompensator.coeffs.Numerator  NumeratorPrototype=[]  FilterStructure=Direct form systolic  SerializationOption=Maximum number of multipliers  NumberOfCycles=2  NumberOfMultipliers=4  SimulateUsing=Code generation  roundingMode=Floor  overflowMode=off  CoefficientsDataTypeStr=fixdt(1,16)  CoefficientsMin=[]  CoefficientsMax=[]  OutputDataTypeStr=Inherit: Same word length as input  OutputMin=[]  OutputMax=[]  ResetInputPort=off  HDLGlobalReset=off
      settings: SourceProductName=DSP System Toolbox  SourceProductBaseCode=DS
  CIC interpolation gain compensation : ArithShift  BitShiftNumber=4  BinPtShiftNumber=double(0)
  Constant : Constant  OutDataTypeStr=boolean  SampleTime=-1
  Constant1 : Constant  OutDataTypeStr=boolean  SampleTime=-1
  Constant2 : Constant  OutDataTypeStr=boolean  SampleTime=-1
  Data Type Conversion : DataTypeConversion  OutDataTypeStr=fixdt(1, 32, 28)  SampleTime=1.30208333333333e-06
  Data Type Conversion1 : DataTypeConversion  OutDataTypeStr=fixdt(1, 32, 28)  SampleTime=2.08333333333333e-05
  Downsample : DownSample  N=double(16)  phase=double(0)  RateOptions=Allow multirate processing
  PipelineRegister : Delay  DelayLength=double(1)  InitialCondition=0  SampleTime=2.08333333333333e-05
  Rate Transition : RateTransition  InitialCondition=double(0)  OutPortSampleTimeOpt=Multiple of input port sample time  OutPortSampleTimeMultiple=1/16
  Rate Transition1 : RateTransition  InitialCondition=double(0)  OutPortSampleTimeOpt=Multiple of input port sample time  OutPortSampleTimeMultiple=1/2048
  Terminator2 : Terminator
  delayMatch{,1..3} (4 alike) : Delay  DelayLength=double(2)  InitialCondition=0  SampleTime=2.08333333333333e-05
  delayMatch4 : Delay  DelayLength=double(32)  InitialCondition=0  SampleTime=1.30208333333333e-06
  delayMatch5 : Delay  DelayLength=double(32)  InitialCondition=0  SampleTime=1.30208333333333e-06
  delayMatch6 : Delay  DelayLength=double(32)  InitialCondition=0  SampleTime=1.30208333333333e-06
  fractional delay DPRAM : hdlsllib/HDL RAMs/Simple Dual Port RAM  ram_size=mp.fractionalDelayAddrSize
      settings: SourceProductName=Simulink  SourceProductBaseCode=SL
  integer delay DPRAM : hdlsllib/HDL RAMs/Simple Dual Port RAM  ram_size=mp.integerDelayAddrSize
      settings: SourceProductName=Simulink  SourceProductBaseCode=SL
  read address generator : Subsystem
  read address generator1 : Subsystem
  split_into_int_and_frac_parts : Subsystem
  write address generator : hdlsllib/Sources/HDL Counter  CountType=Count limited  CountInit=double(0)  CountStep=double(1)  CountMax=double(63)  CountFromType=Initial value  CountFrom=double(0)  CountResetPort=off  CountLoadPort=off  CountEnbPort=off  CountDirPort=off  CountDataType=Unsigned  CountWordLen=6  CountFracLen=0  CountSampTime=2.08333333333333e-05
      settings: SourceProductName=Simulink
  write address generator1 : hdlsllib/Sources/HDL Counter  CountType=Count limited  CountInit=double(0)  CountStep=double(1)  CountMax=double(63)  CountFromType=Initial value  CountFrom=double(0)  CountResetPort=off  CountLoadPort=off  CountEnbPort=off  CountDirPort=off  CountDataType=Unsigned  CountWordLen=6  CountFracLen=0  CountSampTime=1.30208333333333e-06
      settings: SourceProductName=Simulink
  data_out : Outport  VectorParamsAs1DForOutWhenUnconnected=off
  wires:
  Downsample/1 -> PipelineRegister/1
  CIC interpolation gain compensation/1 -> Data Type Conversion/1
  split_into_int_and_frac_parts/1(integer_delay) -> read address generator/2(delay)
  Constant1/1 -> delayMatch6/1
  write address generator1/1 -> delayMatch4/1, delayMatch5/1
  delayMatch5/1 -> fractional delay DPRAM/2
  Constant/1 -> delayMatch3/1
  Constant2/1 -> delayMatch2/1
  write address generator/1 -> delayMatch/1, delayMatch1/1
  delayMatch1/1 -> integer delay DPRAM/2
  delay/1 -> split_into_int_and_frac_parts/1(delay)
  data_in/1 -> integer delay DPRAM/1
  delayMatch3/1 -> CIC interpolation compensator/2
  delayMatch6/1 -> fractional delay DPRAM/3
  delayMatch2/1 -> integer delay DPRAM/3
  Data Type Conversion/1 -> fractional delay DPRAM/1
  Data Type Conversion1/1 -> Rate Transition1/1
  split_into_int_and_frac_parts/2(fractional_delay) -> Rate Transition/1
  read address generator/1(read_addr) -> integer delay DPRAM/4
  read address generator1/1(read_addr) -> fractional delay DPRAM/4
  CIC Interpolation/1 -> CIC interpolation gain compensation/1
  CIC interpolation compensator/2 -> Terminator2/1
  CIC interpolation compensator/1 -> CIC Interpolation/1
  PipelineRegister/1 -> Data Type Conversion1/1
  Rate Transition/1 -> read address generator1/2(delay)
  Rate Transition1/1 -> data_out/1
  fractional delay DPRAM/1 -> Downsample/1
  integer delay DPRAM/1 -> CIC interpolation compensator/1
  delayMatch/1 -> read address generator/1(write_addr)
  delayMatch4/1 -> read address generator1/1(write_addr)
